simulink model "Earth"  (R2024a)
settings: configuration reference "autoCodeSILConfigurationParams" (kept outside this file)
undefined symbols (not defined in the file): Earth, referenceAltitude_m, referenceDecimalYear_years, referenceLatitude_deg, referenceLongitude_deg, WGS84, WMM2020
libraries: aerolibtransform2 x1, aerolibgravity2 x1
settings Model: Creator=jerem  LastModifiedBy=jerem
settings ConfigSetRef: SourceName=autoCodeSILConfigurationParams  SourceLocation=Base Workspace

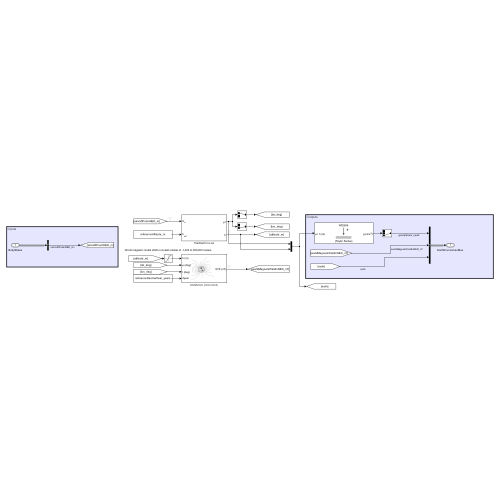
[thumbnail: Simulink's stored preview of the top-level diagram]
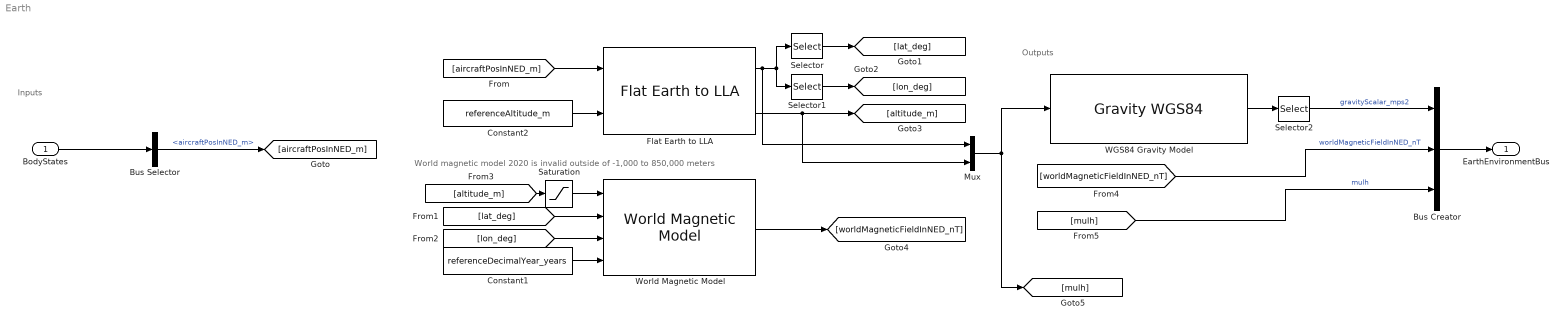
== system Earth ==
  note: World magnetic model 2020 is invalid outside of -1,000 to 850,000 meters
  note: Inputs
  note: Outputs
  BodyStates : Inport  OutDataTypeStr=Bus: BodyStateBus
  Bus Creator : BusCreator  Inputs=3  OutDataTypeStr=Bus: EarthEnvironmentBus  NonVirtualBus=on
  Bus Selector : BusSelector  OutputSignals=aircraftPosInNED_m
  Constant1 : Constant  Value=referenceDecimalYear_years
  Constant2 : Constant  Value=referenceAltitude_m
  Flat Earth to LLA : aerolibtransform2/Flat Earth to LLA  units=Metric (MKS)  ptype=Earth (WGS84)  F=1/298.257223563  R=6378137  refPosPort=off  LL0="[referenceLatitude_deg  referenceLongitude_deg ]"  psi=0
  Mux : Mux  Inputs=2
  Saturation : Saturate  UpperLimit=850000  LowerLimit=-1000
  Selector : Selector  InputPortWidth=2  IndexOptions=Index vector (dialog)  Indices=[1]  OutputSizes=1
  Selector1 : Selector  InputPortWidth=2  IndexOptions=Index vector (dialog)  Indices=[2]  OutputSizes=1
  Selector2 : Selector  InputPortWidth=3  IndexOptions=Index vector (dialog)  Indices=3  OutputSizes=1
  "WGS84 Gravity Model  " : GravityWGS84  action=None
  World Magnetic Model : aerolibgravity2/World Magnetic Model  model=WMM2020 (2020-2025)  customFile='WMM2020.COF'  units=Metric (MKS)  time_in=on  month=January  day=1  year=2024  action=Error  h_out=off  dec_out=off  inc_out=off  ti_out=off
  EarthEnvironmentBus : Outport  OutDataTypeStr=Bus: EarthEnvironmentBus
  wires:
  "WGS84 Gravity Model  "/1 -> Selector2/1
  Bus Creator/1 -> EarthEnvironmentBus/1
  BodyStates/1 -> Bus Selector/1
  Constant1/1 -> World Magnetic Model/4
  Bus Selector/1 -> [aircraftPosInNED_m]  "<aircraftPosInNED_m>"
  [aircraftPosInNED_m] -> Flat Earth to LLA/1
  Flat Earth to LLA/2 -> Mux/2, [altitude_m]
  Flat Earth to LLA/1 -> Mux/1, Selector/1, Selector1/1
  Selector/1 -> [lat_deg]
  Selector1/1 -> [lon_deg]
  [lon_deg] -> World Magnetic Model/3
  [lat_deg] -> World Magnetic Model/2
  [altitude_m] -> Saturation/1
  Constant2/1 -> Flat Earth to LLA/2
  World Magnetic Model/1 -> [worldMagneticFieldInNED_nT]
  [worldMagneticFieldInNED_nT] -> Bus Creator/2  "worldMagneticFieldInNED_nT"
  Saturation/1 -> World Magnetic Model/1
  Mux/1 -> [mulh], "WGS84 Gravity Model  "/1
  Selector2/1 -> Bus Creator/1  "gravityScalar_mps2"
  [mulh] -> Bus Creator/3  "mulh"
